simulink model "Model_Step"  (R2015a)
settings: Solver=ode3  StartTime=0.0  StopTime=10  FixedStep=0.01  RelTol=1e-3
undefined symbols (not defined in the file or in its folder): sigbuilder_block
libraries: fuzblock x1
settings Model: Creator=Φίλιππος  LastModifiedBy=ALKATRAZ
settings ConfigComp: Description=Design Verifier Custom Configuration Component  DVMaxTestCaseSteps=500  DVTestSuiteOptimization=CombinedObjectives (Nonlinear Extended)

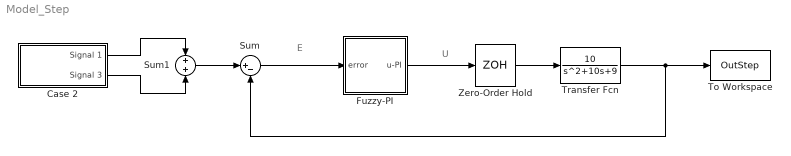
== system Model_Step ==
  note: U
  note: E
  Case 2 : Subsystem  Tag=STV Subsys  LoadFcn=sigbuilder_block('load');  StartFcn=sigbuilder_block('start');  StopFcn=sigbuilder_block('stop');  ClipboardFcn=sigbuilder_block('clipboard');  mask(Sigbuilder block){}
      mask help: Simulink:masks:SigbuilderBlock_MD
      mask init:
      | if ~strcmp(get_param(bdroot(gcbh),'SimulationStatus'),'stopped') tuvar = sigbuilder_block('maskInit'); end
      settings: CopyFcn=sigbuilder_block('copy');  DeleteFcn=sigbuilder_block('delete');  ModelCloseFcn=sigbuilder_block('modelClose');  PreSaveFcn=sigbuilder_block('preSave');  PauseFcn=sigbuilder_block('pause');  ContinueFcn=sigbuilder_block('continue');  NameChangeFcn=sigbuilder_block('namechange');  OpenFcn=sigbuilder_block('open',[437.6 199.2 550.4 400 ]);  CloseFcn=sigbuilder_block('close');
      mask Display: plot(0, 0, 100, 100,[2, 2, 32, 32, 2], [68, 8, 8, 68, 68],[32, 2], [38, 38], [32, 19, 2],[53, 60, 44], [32, 17, 17, 2],[16, 16, 31, 31]);txt = getActiveGroup(gcbh);text(2, 100, txt,'verticalAlignment', 'top');
  Fuzzy-PI : Subsystem
  Sum : Sum  Inputs=|+-
  Sum1 : Sum
  To Workspace : ToWorkspace  VariableName=OutStep  SaveFormat=Timeseries  SampleTime=-1
  Transfer Fcn : TransferFcn  Numerator=[10]  Denominator=[1 10 9]
  Zero-Order Hold : ZeroOrderHold  SampleTime=0.01
  wires:
  Zero-Order Hold/1 -> Transfer Fcn/1
  Transfer Fcn/1 -> To Workspace/1, Sum/2
  Fuzzy-PI/1(u-PI) -> Zero-Order Hold/1
  Sum/1 -> Fuzzy-PI/1(error)
  Case 2/1(Signal 1) -> Sum1/1
  Sum1/1 -> Sum/1
  Case 2/2(Signal 3) -> Sum1/2

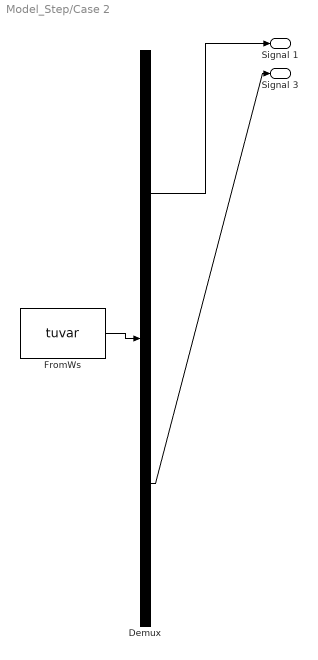
== system Model_Step/Case 2 ==
  Demux : Demux  Tag=STV Demux  Outputs=2
  FromWs : FromWorkspace  Tag=STV FromWs  VariableName=tuvar  SampleTime=0
      SigBuilderData=|
      | common.afterFinalStr = 'Extrapolate'
      | common.sampleTime = 0
      | dataSet.timeRange = [0 10]
      | dataSet.name = 'Group 1'
      | sbobj.Groups.Name = 'Group 1'
      | sbobj.Groups.Signals(1).Name = 'Signal 1'
      | sbobj.Groups.Signals(1).XData = [0 4 4 10]
      | sbobj.Groups.Signals(1).YData = [60 60 20 20]
      | sbobj.Groups.Signals(2).Name = 'Signal 3'
      | sbobj.Groups.Signals(2).XData = [0 8 8 10]
      | sbobj.Groups.Signals(2).YData = [0 0 20 20]
  Signal 1 : Outport  Tag=STV Outport
  Signal 3 : Outport  Tag=STV Outport  Port=2
  wires:
  Demux/1 -> Signal 1/1
  FromWs/1 -> Demux/1
  Demux/2 -> Signal 3/1

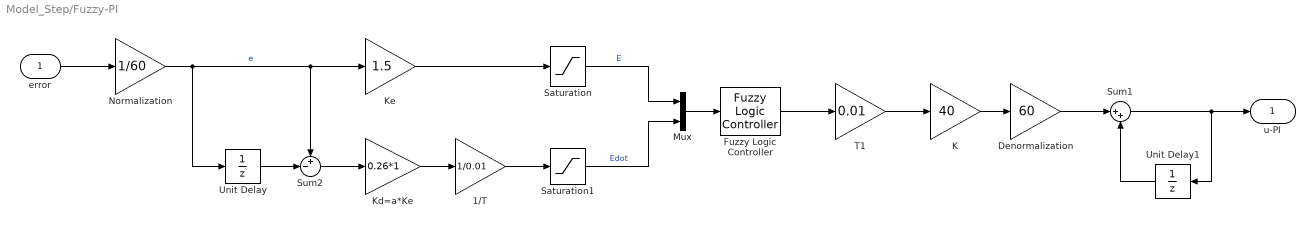
== system Model_Step/Fuzzy-PI ==
  error : Inport
  1/T : Gain  Gain=1/0.01
  Denormalization : Gain  Gain=60
  Fuzzy Logic Controller : fuzblock/Fuzzy Logic  Controller  fis='FuzzyController.fis'
  K : Gain  Gain=40
  Kd=a*Ke : Gain  Gain=0.26*1
  Ke : Gain  Gain=1.5
  Mux : Mux  Inputs=2
  Normalization : Gain  Gain=1/60
  Saturation : Saturate  UpperLimit=1  LowerLimit=-1
  Saturation1 : Saturate  UpperLimit=1  LowerLimit=-1
  Sum1 : Sum  Inputs=|++
  Sum2 : Sum  Inputs=+-|
  T1 : Gain  Gain=0.01
  Unit Delay : UnitDelay  SampleTime=-1
  Unit Delay1 : UnitDelay  SampleTime=-1
  u-PI : Outport
  wires:
  error/1 -> Normalization/1
  Normalization/1 -> Unit Delay/1, Sum2/1, Ke/1  "e"
  Unit Delay/1 -> Sum2/2
  Ke/1 -> Saturation/1
  Kd=a*Ke/1 -> 1/T/1
  1/T/1 -> Saturation1/1
  Saturation/1 -> Mux/1  "E"
  Saturation1/1 -> Mux/2  "Edot"
  Mux/1 -> Fuzzy Logic Controller/1
  Fuzzy Logic Controller/1 -> T1/1
  T1/1 -> K/1
  K/1 -> Denormalization/1
  Denormalization/1 -> Sum1/1
  Sum1/1 -> Unit Delay1/1, u-PI/1
  Unit Delay1/1 -> Sum1/2
  Sum2/1 -> Kd=a*Ke/1
